simulink model "Model"  (R2017a)
settings: Solver=VariableStepAuto  StartTime=0.0  StopTime=inf  RelTol=1e-3
model workspace (MAT data in the model file):
  throttleOutput = 1000
undefined symbols (not defined in the file or in its folder): magnitude
libraries: simulink x1, slident x1
settings Model: Creator=Ray  LastModifiedBy=Ray

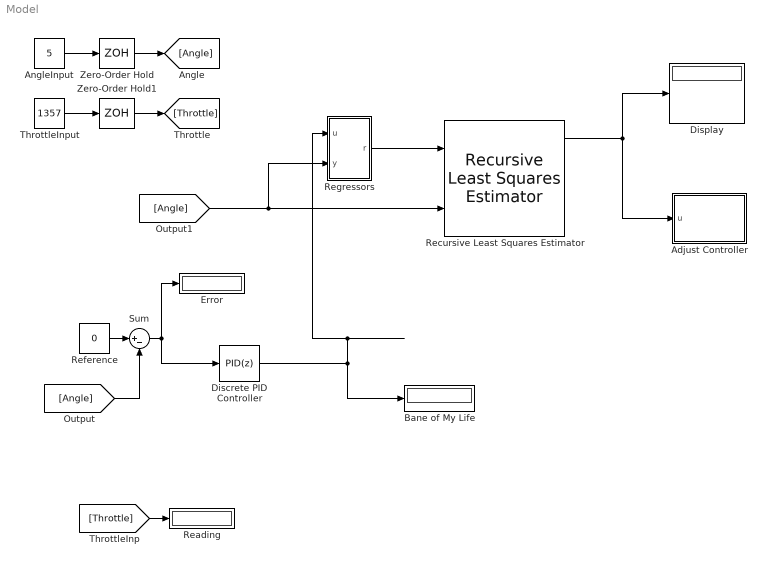
== system Model ==
  Adjust Controller : MATLAB Function  TreatAsAtomicUnit=on
  AngleInput : Constant  Value=5  SampleTime=0.1
  Bane of My Life : Display
  Discrete PID Controller : simulink/Continuous/PID Controller  Controller=PID  TimeDomain=Discrete-time  SampleTime=-1  IntegratorMethod=Forward Euler  FilterMethod=Forward Euler  Form=Parallel  UseFilter=on  ControllerParametersSource=internal  P=8  I=2.7  D=0  N=100  InitialConditionSource=internal  InitialConditionForIntegrator=0  InitialConditionForFilter=0  ExternalReset=none  LimitOutput=on  UpperSaturationLimit=2000  LowerSaturationLimit=1000  LinearizeAsGain=off  AntiWindupMode=none  Kb=1  TrackingMode=off  Kt=1  PParamMin=[]  PParamMax=[]  IParamMin=[]  IParamMax=[]  DParamMin=[]  DParamMax=[]  NParamMin=[]  NParamMax=[]  KbParamMin=[]  KbParamMax=[]  KtParamMin=[]  KtParamMax=[]  POutMin=[]  POutMax=[]  IOutMin=[]  IOutMax=[]  DOutMin=[]  DOutMax=[]  NOutMin=[]  NOutMax=[]  KbOutMin=[]  KbOutMax=[]  KtOutMin=[]  KtOutMax=[]  IntegratorOutMin=[]  IntegratorOutMax=[]  FilterOutMin=[]  FilterOutMax=[]  SumOutMin=[]  SumOutMax=[]  SumI1OutMin=[]  SumI1OutMax=[]  SumI2OutMin=[]  SumI2OutMax=[]  SumI3OutMin=[]  SumI3OutMax=[]  SumDOutMin=[]  SumDOutMax=[]  SaturationOutMin=[]  SaturationOutMax=[]  IntegratorContinuousStateAttributes=''  IntegratorStateMustResolveToSignalObject=off  IntegratorRTWStateStorageClass=Auto  FilterContinuousStateAttributes=''  FilterStateMustResolveToSignalObject=off  FilterRTWStateStorageClass=Auto  DifferentiatorICPrevScaledInput=0  DifferentiatorOutMin=[]  DifferentiatorOutMax=[]  InitialConditionSetting=State (most efficient)
  Display : Display
  Error : Display
  Reading : Display
  Recursive Least Squares Estimator : slident/Estimators/Recursive Least Squares Estimator  InitialEstimateSource=None  InitialParameterData=5  P0=1  EstimationMethod=Forgetting Factor  AdaptationParameter=1-2e-4  NormalizationBias=eps  OutputError=on  OutputP=on  AddEnablePort=off  Ts=0.1
      settings: SourceProductName=System Identification Toolbox  SourceProductBaseCode=ID
  Reference : Constant  Value=0
  Regressors : Subsystem
  Sum : Sum  Inputs=|+-
  ThrottleInput : Constant  Value=1357  SampleTime=0.1
  Zero-Order Hold : ZeroOrderHold  SampleTime=0.1
  Zero-Order Hold1 : ZeroOrderHold  SampleTime=0.1
  wires:
  Regressors/1(r) -> Recursive Least Squares Estimator/1
  AngleInput/1 -> Zero-Order Hold/1
  Recursive Least Squares Estimator/1 -> Adjust Controller/1(u), Display/1
  ThrottleInput/1 -> Zero-Order Hold1/1
  Reference/1 -> Sum/1
  Sum/1 -> Discrete PID Controller/1, Error/1
  Zero-Order Hold/1 -> [Angle]
  [Angle] -> Sum/2
  [Angle] -> Recursive Least Squares Estimator/2, Regressors/2(y)
  Zero-Order Hold1/1 -> [Throttle]
  [Throttle] -> Reading/1
  Discrete PID Controller/1 -> Regressors/1(u), Bane of My Life/1

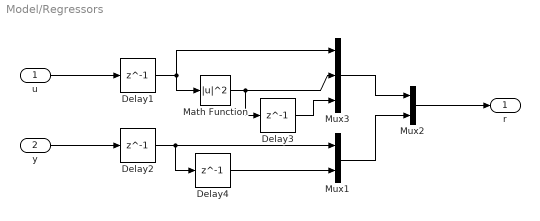
== system Model/Regressors ==
  u : Inport
  y : Inport  Port=2
  Delay1 : Delay  DelayLength=1  InitialCondition=1  SampleTime=0.1
  Delay2 : Delay  DelayLength=1  InitialCondition=2  SampleTime=0.1
  Delay3 : Delay  DelayLength=1  InitialCondition=1  SampleTime=0.1
  Delay4 : Delay  DelayLength=1  InitialCondition=2  SampleTime=0.1
  Math Function : Math  Operator=magnitude^2  SaturateOnIntegerOverflow=on
  Mux1 : Mux  Inputs=2
  Mux2 : Mux  Inputs=2
  Mux3 : Mux  Inputs=3
  r : Outport
  wires:
  u/1 -> Delay1/1
  Mux2/1 -> r/1
  Delay1/1 -> Mux3/1, Math Function/1
  y/1 -> Delay2/1
  Mux3/1 -> Mux2/1
  Delay2/1 -> Delay4/1, Mux1/1
  Math Function/1 -> Delay3/1, Mux3/2
  Delay3/1 -> Mux3/3
  Delay4/1 -> Mux1/2
  Mux1/1 -> Mux2/2

== matlab function Model/Adjust Controller ==
  data: u input
function fcn(u)
    
end
